simulink model "initial_simulation_forward"  (R2018b)
settings: Solver=VariableStepAuto  StartTime=0.0  StopTime=10.0  RelTol=1e-3
settings Model: Creator=299792458  LastModifiedBy=ali

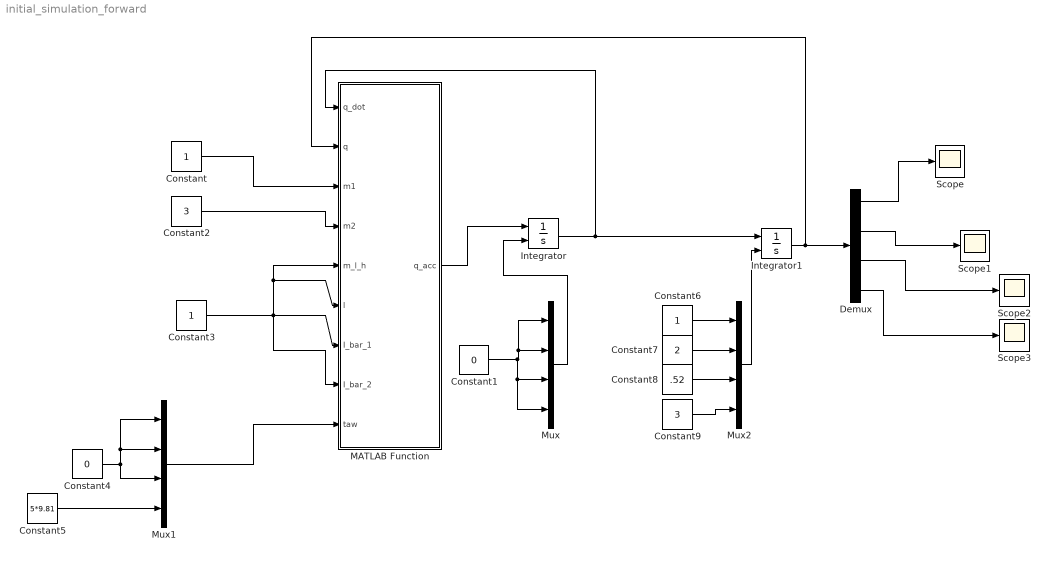
== system initial_simulation_forward ==
  Constant : Constant
  Constant1 : Constant  Value=0
  Constant2 : Constant  Value=3
  Constant3 : Constant
  Constant4 : Constant  Value=0
  Constant5 : Constant  Value=5*9.81
  Constant6 : Constant
  Constant7 : Constant  Value=2
  Constant8 : Constant  Value=.52
  Constant9 : Constant  Value=3
  Demux : Demux
  Integrator : Integrator  InitialConditionSource=external  InitialCondition=[0;0;0;0]
  Integrator1 : Integrator  InitialConditionSource=external  InitialCondition=[0;0;0;0]
  MATLAB Function : MATLAB Function  TreatAsAtomicUnit=on
  Mux : Mux
  Mux1 : Mux
  Mux2 : Mux
  Scope{,1..3} (4 alike) : Scope
  wires:
  MATLAB Function/1(q_acc) -> Integrator/1
  Integrator/1 -> MATLAB Function/1(q_dot), Integrator1/1
  Integrator1/1 -> MATLAB Function/2(q), Demux/1
  Constant/1 -> MATLAB Function/3(m1)
  Constant1/1 -> Mux/4, Mux/3, Mux/2, Mux/1
  Mux/1 -> Integrator/2
  Constant2/1 -> MATLAB Function/4(m2)
  Constant3/1 -> MATLAB Function/8(I_bar_2), MATLAB Function/7(I_bar_1), MATLAB Function/6(l), MATLAB Function/5(m_l_h)
  Constant4/1 -> Mux1/1, Mux1/2, Mux1/3
  Mux1/1 -> MATLAB Function/9(taw)
  Mux2/1 -> Integrator1/2
  Constant6/1 -> Mux2/1
  Constant7/1 -> Mux2/2
  Constant8/1 -> Mux2/3
  Constant9/1 -> Mux2/4
  Demux/1 -> Scope/1
  Demux/2 -> Scope1/1
  Demux/3 -> Scope2/1
  Demux/4 -> Scope3/1
  Constant5/1 -> Mux1/4

== matlab function initial_simulation_forward/MATLAB Function ==
  data: q_dot input; q input; m1 input; q_acc output; m2 input; m_l_h input; l input; I_bar_1 input; I_bar_2 input; taw input
function q_acc = fcn(q_dot, q,m1,m2,m_l_h,l,I_bar_1,I_bar_2,taw)
% q=[r1;r2;theta;z];
% q_dot=[r1_d;r2_d;theta_d;z_d];
g=9.81;
M_mat =[m1,0,0,0
        0, m2,0,0
        0,  0, (7*m_l_h*l^2)/27 + m1*q(1,1)^2 + m2*q(2,1)^2 + I_bar_1 + I_bar_2 ,               0
        0,  0,0, m1 + m2 + m_l_h];

G_vec=[0
    0
    0
    g*(m1 + m2 + m_l_h)];

C_mat=[0,0,-m1*q(1,1)*q_dot(3,1), 0
    0,0, -m2*q(2,1)*q_dot(3,1), 0
    2*m1*q(1,1)*q_dot(3,1), 2*m2*q(2,1)*q_dot(3,1), 0, 0
    0,0, 0, 0];
M_mat_inv=inv(M_mat);

q_acc=M_mat_inv*(taw-C_mat*q_dot-G_vec);
end
